simulink model "eem441"  (Simulink 7.0)
settings: Solver=ode45  StartTime=0.0  StopTime=10.0  RelTol=1e-3
settings Model: Creator=PACKARDBELL  LastModifiedBy=user

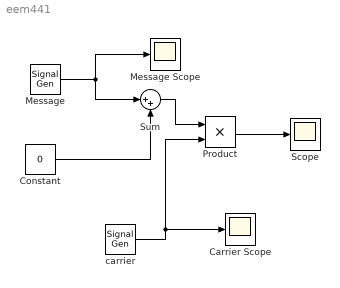
== system eem441 ==
  Carrier Scope : Scope
      settings: SaveName=ScopeData2
  Constant : Constant  Value=0  OutDataType=sfix(16)  OutScaling=2^0
  Message : SignalGenerator  Frequency=167
  Message Scope : Scope
  Product : Product  OutDataType=sfix(16)  OutScaling=2^0  SampleTime=.001  RndMeth=Zero
  Scope : Scope
  Sum : Sum  Inputs=|++  OutDataType=sfix(16)  OutScaling=2^0
  carrier : SignalGenerator  Frequency=100
  wires:
  Message/1 -> Sum/1, Message Scope/1
  Constant/1 -> Sum/2
  Sum/1 -> Product/1
  carrier/1 -> Product/2, Carrier Scope/1
  Product/1 -> Scope/1
